simulink subsystem "saturation"  (R2025b)
settings: Solver=VariableStepAuto  StartTime=0.0  StopTime=10.0  RelTol=1e-3
libraries: simulink x1
settings Model: Creator=maxhu  LastModifiedBy=maxhu

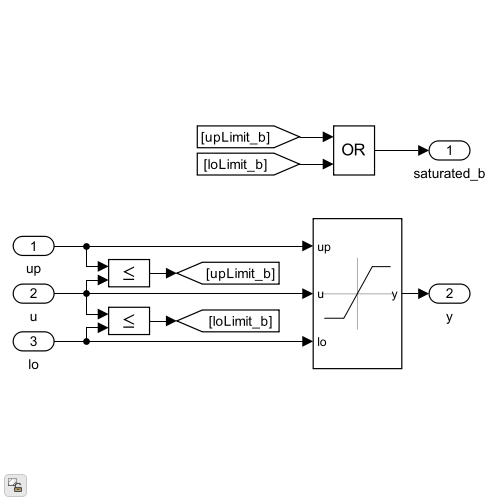
[thumbnail: Simulink's stored preview of the top-level diagram]
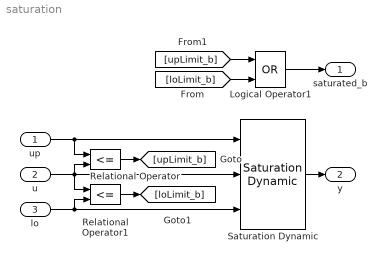
== system saturation ==
  up : Inport
  u : Inport  Port=2
  lo : Inport  Port=3
  Logical Operator1 : Logic  Operator=OR  AllPortsSameDT=off  OutDataTypeStr=boolean
  Relational Operator : RelationalOperator  Operator=<=  OutDataTypeStr=boolean  RndMeth=Simplest  InputSameDT=off
  Relational Operator1 : RelationalOperator  Operator=<=  OutDataTypeStr=boolean  RndMeth=Simplest  InputSameDT=off
  Saturation Dynamic : simulink/Discontinuities/Saturation Dynamic  OutMin=[]  OutMax=[]  OutDataTypeStr=Inherit: Same as second input  OutDataType=fixdt(1, 16)  OutScaling=2^-10  DoSatur=off
  saturated_b : Outport
  y : Outport  Port=2
  wires:
  u/1 -> Relational Operator/2, Saturation Dynamic/2, Relational Operator1/1
  up/1 -> Relational Operator/1, Saturation Dynamic/1
  lo/1 -> Relational Operator1/2, Saturation Dynamic/3
  Saturation Dynamic/1 -> y/1
  Logical Operator1/1 -> saturated_b/1
  Relational Operator/1 -> [upLimit_b]
  Relational Operator1/1 -> [loLimit_b]
  [upLimit_b] -> Logical Operator1/1
  [loLimit_b] -> Logical Operator1/2
